simulink library "hdlsllib"  (R2019a)
settings: Solver=ode45  StartTime=0.0  StopTime=10.0  RelTol=1e-3  EnableMultiTasking=on
values from neighbouring files (symbols this model uses):
  freerun = strcmp(get_param(blk, 'CountType'), 'Free running')    [hdlblkmask_counter.m]
  maxval_sc = countrange(2)    [hdlblkmask_counter.m]
  samptime = -1    [hdlblkmask_counter.m]
undefined symbols (not defined in the file or in its folder): a, b, c, Dialog, DiscIntNeverNeededParam, Floor, HDLStatusEnum, jsin, magnitude, message, Newton, NumBits1, NumBits2, Raphson, Slope1, Slope2
libraries: simulink x70, $bdroot x5, hdlmdlgenlib x1, hdlsllib_helper x1
(part 3 of 3)

== matlab function hdlsllib/HDL Operations/Deserializer1D/IntToEnumConverter ==
  data: dataIn input; deserializer_PostProcessed output; dataOut input
function deserializer_PostProcessed = fcn(dataIn, dataOut)
%#codegen
% added to support enum dataIn
if(coder.isenum(dataIn))  %is enum dataIn, convert dataOut back to enum
    EnumClassIn = class(dataIn);
    fh = str2func(EnumClassIn);
    deserializer_PostProcessed = fh(dataOut);
else
    deserializer_PostProcessed = dataOut;
end

== matlab function hdlsllib/Logic and Bit Operations/Bit Slice/bit_slice ==
  data: u input; y output; lidx parameter; ridx parameter
function y = fcn(u, lidx, ridx)
%#codegen

y = bitsliceget(cast_to_fi(u), lidx+1, ridx+1);

== matlab function hdlsllib/Logic and Bit Operations/Bit Reduce/bit_reduce ==
  data: u input; y output; mode parameter
function y = fcn(u,mode)
%#codegen

switch mode
    case 1
        y = bitandreduce(cast_to_fi(u));        
    case 2
        y = bitorreduce(cast_to_fi(u));
    case 3
        y = bitxorreduce(cast_to_fi(u));
    otherwise             
        y = cast_to_fi(u);
end

== matlab function hdlsllib/Logic and Bit Operations/Bit Rotate/bit_rotate ==
  data: u input; y output; mode parameter; N parameter
function y = fcn(u, mode, N)
%#codegen

switch mode
    case 1
        y = bitrol(cast_to_fi(u), N);
    case 2
        y = bitror(cast_to_fi(u), N);
    otherwise
        y = u;
end

== matlab function hdlsllib/Logic and Bit Operations/Bit Shift/bit_shift ==
  data: u input; y output; mode parameter; N parameter
function y = fcn(u, mode, N)
%#codegen

switch mode
    case 1
        y = bitsll(cast_to_fi(u), N);
    case 2
        y = bitsrl(cast_to_fi(u), N);
    case 3
        y = bitsra(cast_to_fi(u), N);
    otherwise
        y = cast_to_fi(u);
end
